simulink model "sysgen_oversample2x_2samples_per_clock"  (R2016b)
settings: Solver=VariableStepAuto  StartTime=0.0  StopTime=samples_per_channel*number_channels  RelTol=1e-3
PreLoadFcn:
  | setup
undefined symbols (not defined in the file or in its folder): j
libraries: xbsIndex_r4 x355, dspsigops x2, hdlsllib x2
(part 3 of 3)

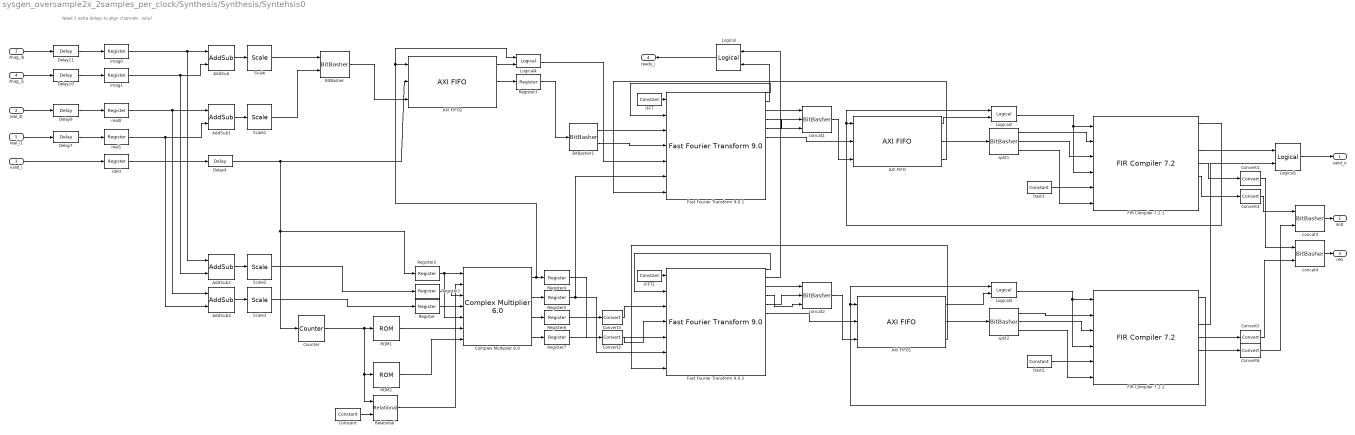
== system sysgen_oversample2x_2samples_per_clock/Synthesis/Synthesis/Syntehsis0 ==
  note: Need 2 extra delays to align channels - why?
  imag_i0 : Inport
  real_i0 : Inport  Port=2
  valid_i : Inport  Port=3
  imag_i1 : Inport  Port=4
  real_i1 : Inport  Port=5
  AXI FIFO : xbsIndex_r4/AXI FIFO  input_depth_axis=16  actual_fifo_depth_label=18  enable_tdata=on  enable_tdest=off  enable_tstrb=off  enable_tready=on  enable_tid=off  enable_tuser=off  enable_tkeep=off  enable_tlast=off  has_aresetn=off  enable_data_counts_axis=off  fifo_implementation_type_axis=Common Clock Block RAM  trim_axipin_name=on  programmable_full_type_axis=Full  full_threshold_assert_value_axis=0  programmable_empty_type_axis=Empty  empty_threshold_assert_value_axis=1022  underflow_flag_axi=0  underflow_sense_axi=Active High  overflow_flag_axi=0  overflow_sense_axi=Active High  block_type=axi_fifo
  AXI FIFO1 : xbsIndex_r4/AXI FIFO  input_depth_axis=16  actual_fifo_depth_label=18  enable_tdata=on  enable_tdest=off  enable_tstrb=off  enable_tready=on  enable_tid=off  enable_tuser=off  enable_tkeep=off  enable_tlast=off  has_aresetn=off  enable_data_counts_axis=off  fifo_implementation_type_axis=Common Clock Block RAM  trim_axipin_name=on  programmable_full_type_axis=Full  full_threshold_assert_value_axis=0  programmable_empty_type_axis=Empty  empty_threshold_assert_value_axis=1022  underflow_flag_axi=0  underflow_sense_axi=Active High  overflow_flag_axi=0  overflow_sense_axi=Active High  block_type=axi_fifo
  AXI FIFO2 : xbsIndex_r4/AXI FIFO  input_depth_axis=16  actual_fifo_depth_label=18  enable_tdata=on  enable_tdest=off  enable_tstrb=off  enable_tready=on  enable_tid=off  enable_tuser=off  enable_tkeep=off  enable_tlast=off  has_aresetn=off  enable_data_counts_axis=off  fifo_implementation_type_axis=Common Clock Block RAM  trim_axipin_name=on  programmable_full_type_axis=Full  full_threshold_assert_value_axis=0  programmable_empty_type_axis=Empty  empty_threshold_assert_value_axis=1022  underflow_flag_axi=0  underflow_sense_axi=Active High  overflow_flag_axi=0  overflow_sense_axi=Active High  block_type=axi_fifo
  AddSub : xbsIndex_r4/AddSub  mode=Addition  use_carryin=off  use_carryout=off  en=off  latency=2  precision=Full  arith_type="Signed  (2's comp)"  n_bits=17  bin_pt=15  quantization=Truncate  overflow=Saturate  use_behavioral_HDL=on  hw_selection=Fabric  pipelined=off  dbl_ovrd=off  block_type=addsub
  AddSub1 : xbsIndex_r4/AddSub  mode=Addition  use_carryin=off  use_carryout=off  en=off  latency=2  precision=Full  arith_type="Signed  (2's comp)"  n_bits=17  bin_pt=15  quantization=Truncate  overflow=Saturate  use_behavioral_HDL=on  hw_selection=Fabric  pipelined=off  dbl_ovrd=off  block_type=addsub
  AddSub2 : xbsIndex_r4/AddSub  mode=Subtraction  use_carryin=off  use_carryout=off  en=off  latency=2  precision=Full  arith_type="Signed  (2's comp)"  n_bits=17  bin_pt=15  quantization=Truncate  overflow=Saturate  use_behavioral_HDL=on  hw_selection=Fabric  pipelined=off  dbl_ovrd=off  block_type=addsub
  AddSub4 : xbsIndex_r4/AddSub  mode=Subtraction  use_carryin=off  use_carryout=off  en=off  latency=2  precision=Full  arith_type="Signed  (2's comp)"  n_bits=17  bin_pt=15  quantization=Truncate  overflow=Saturate  use_behavioral_HDL=on  hw_selection=Fabric  pipelined=off  dbl_ovrd=off  block_type=addsub
  BitBasher : xbsIndex_r4/BitBasher  bitexpr=out = {30'b0, im, re}  display_expr=off  sr_1=out  arith_type1=Unsigned  bin_pt1=0  sr_2=2  arith_type2=Unsigned  bin_pt2=0  sr_3=3  arith_type3=Unsigned  bin_pt3=0  sr_4=4  arith_type4=Unsigned  bin_pt4=0  dbl_ovrd=off  block_type=bitbasher
  BitBasher1 : xbsIndex_r4/BitBasher  bitexpr=|  display_expr=off  sr_1=im  arith_type1="Signed  (2's comp)"  bin_pt1=16  sr_2=re  arith_type2="Signed  (2's comp)"  bin_pt2=16  sr_3=3  arith_type3=Unsigned  bin_pt3=0  sr_4=4  arith_type4=Unsigned  bin_pt4=0  dbl_ovrd=off  block_type=bitbasher
      | im = {in[33:17]}
      | re = {in[16:0]}
  "Complex Multiplier 6.0 " : xbsIndex_r4/Complex Multiplier 6.0   hasatlast=on  hasatuser=off  atuserwidth=1  hasbtlast=off  hasbtuser=off  btuserwidth=1  multtype=Use_Mults  optimizegoal=Resources  flowcontrol=NonBlocking  outputwidth=19  roundmode=Truncate  hasctrltlast=off  hasctrltuser=off  ctrltuserwidth=1  outtlastbehv=Null  latencyconfig=Automatic  minimumlatency=37  aclken=off  aresetn=off  trim_axipin_name=on  simulation_type=hybrid_sim  simulation_model=sysgen:cmpy_v6_0  data_path_portlist={ 's_axis_a_tdata_real', 's_axis_a_tdata_imag', 's_axis_b_tdata_real', 's_axis_b_tdata_imag', 's_axis_ctrl_tdata_rounding_bit', 'm_axis_dout_tdata_real', 'm_axis_dout_tdata_imag' }  aportwidth=63  bportwidth=63  ip_name=Complex Multiplier  ip_version=6.0  dsptool_ready=true  ipcore_usecache=true  ipcore_useipmodelcache=true  ipcore_verbose=false  ipcore_latency_parameter='minimumlatency'  wrapper_available=true  port_translation_map={ 'aclken' => 'en', 'aresetn' => 'rst'}  block_type=cmpy_v6_0
  Constant : xbsIndex_r4/Constant  const=7  gui_display_data_type=Fixed-point  arith_type=Unsigned  n_bits=3  bin_pt=0  preci_type=Single  exp_width=8  frac_width=24  explicit_period=off  period=1  equ=P=C  opselect=C  inp2=PCIN>>17  opr=+  inp1=P  carry=CIN  dbl_ovrd=off  block_type=constant
  Convert{1,4..6} (4 alike) : xbsIndex_r4/Convert  gui_display_data_type=Fixed-point  arith_type="Signed  (2's comp)"  n_bits=16  bin_pt=15  float_type=Single  exp_bits=8  fraction_bits=24  quantization=Truncate  overflow=Wrap  en=off  latency=1  pipeline=off  dbl_ovrd=off  block_type=convert
  Convert2 : xbsIndex_r4/Convert  gui_display_data_type=Fixed-point  arith_type="Signed  (2's comp)"  n_bits=17  bin_pt=16  float_type=Single  exp_bits=8  fraction_bits=24  quantization=Truncate  overflow=Wrap  en=off  latency=0  pipeline=off  dbl_ovrd=off  block_type=convert
  Convert3 : xbsIndex_r4/Convert  gui_display_data_type=Fixed-point  arith_type="Signed  (2's comp)"  n_bits=17  bin_pt=16  float_type=Single  exp_bits=8  fraction_bits=24  quantization=Truncate  overflow=Wrap  en=off  latency=0  pipeline=off  dbl_ovrd=off  block_type=convert
  Counter : xbsIndex_r4/Counter  cnt_type=Free Running  cnt_to=Inf  operation=Up  start_count=0  cnt_by_val=1  arith_type=Unsigned  n_bits=3  bin_pt=0  load_pin=off  rst=off  en=on  explicit_period=on  period=2  use_behavioral_HDL=off  implementation=Fabric  dbl_ovrd=off  block_type=counter
  Delay{4,7,9..11} (5 alike) : xbsIndex_r4/Delay  rst=off  infoeditControl=Selection of Reset will increase slice count due to use of real FFs and instead of SRLs  en=off  latency=2  reg_retiming=off  dbl_ovrd=off  block_type=delay
  FIR Compiler 7.2 1 : xbsIndex_r4/FIR Compiler 7.2   coefficientvector=synthesis_coefficients1  coefficient_sets=8  coefficient_reload=off  filter_type=Single_Rate  rate_change_type=Integer  interpolation_rate=1  decimation_rate=1  zero_pack_factor=1  channel_sequence=Basic  number_channels=8  pattern_list='P4-0,P4-1,P4-2,P4-3,P4-4'  number_paths=2  ratespecification=Output_Sample_Period  sampleperiod=1  hardwareoversamplingrate=1  coefficient_sign=Signed  quantization=Quantize_Only  coefficient_width=25  bestprecision=on  coefficient_fractional_bits=28  coefficient_structure=Inferred  output_rounding_mode=Convergent_Rounding_to_Even  output_width=19  filter_architecture=Systolic_Multiply_Accumulate  optimization_goal=Area  optimization_list='None'  data_buffer_type=Automatic  coefficient_buffer_type=Automatic  input_buffer_type=Automatic  output_buffer_type=Automatic  preference_for_other_storage=Automatic  multi_column_support=Automatic  columnconfig='16'  inter_column_pipe_length=4  data_has_tlast=Not_Required  m_data_has_tready=off  s_data_has_fifo=off  s_data_has_tuser=Not_Required  m_data_has_tuser=Not_Required  s_config_sync_mode=On_Vector  s_config_method=By_Channel  num_reload_slots=1  has_aclken=off  has_aresetn=off  infoeditControl=ARESETn must be asserted for a minimum of 2 cycles  reset_data_vector=on  trim_axipin_name=on  simulation_type=hybrid_sim  simulation_model=sysgen:xfirv7_2_cmodel  data_path_portlist={ 's_axis_data_tdata', 'm_axis_data_tdata' }  passband_min=0.0  passband_max=0.5  stopband_min=0.5  stopband_max=1.0  filter_selection=1  gui_behaviour='Sysgen_GUI'  data_sign=Signed  data_width=16  data_fractional_bits=0  data_tuser_width=1  wrapper_available=true  ip_wrap_arbitrary_binary_point=true  ip_name=FIR Compiler  ip_version=7.2  dsptool_ready=true  ipcore_usecache=true  ipcore_useipmodelcache=true  port_translation_map={ 'aclken' => 'en', 'aresetn' => 'rst' }  run_core_at_system_period=true  ipcore_xco_need_fpga_part=true  block_type=fir_compiler_v7_2
      settings: infoedit=Maximum Possible : Maximizes oversampling rate. Abstracted input handshake (no s_data_tvalid) and automatic rate propagation.<br>Hardware Oversampling Rate : Specifies oversampling rate relative to the input sample period. Abstracted input handshake (no s_data_tvalid) and automatic rate propagation.<br>Input/Output Sample Period : Specifies absolute oversampling rate. No input handshake abstraction (exposes s_data_tvalid) and no rate propagation.
  FIR Compiler 7.2 2 : xbsIndex_r4/FIR Compiler 7.2   coefficientvector=synthesis_coefficients2  coefficient_sets=8  coefficient_reload=off  filter_type=Single_Rate  rate_change_type=Integer  interpolation_rate=1  decimation_rate=1  zero_pack_factor=1  channel_sequence=Basic  number_channels=8  pattern_list='P4-0,P4-1,P4-2,P4-3,P4-4'  number_paths=2  ratespecification=Output_Sample_Period  sampleperiod=1  hardwareoversamplingrate=1  coefficient_sign=Signed  quantization=Quantize_Only  coefficient_width=25  bestprecision=on  coefficient_fractional_bits=28  coefficient_structure=Inferred  output_rounding_mode=Convergent_Rounding_to_Even  output_width=19  filter_architecture=Systolic_Multiply_Accumulate  optimization_goal=Area  optimization_list='None'  data_buffer_type=Automatic  coefficient_buffer_type=Automatic  input_buffer_type=Automatic  output_buffer_type=Automatic  preference_for_other_storage=Automatic  multi_column_support=Automatic  columnconfig='16'  inter_column_pipe_length=4  data_has_tlast=Not_Required  m_data_has_tready=off  s_data_has_fifo=off  s_data_has_tuser=Not_Required  m_data_has_tuser=Not_Required  s_config_sync_mode=On_Vector  s_config_method=By_Channel  num_reload_slots=1  has_aclken=off  has_aresetn=off  infoeditControl=ARESETn must be asserted for a minimum of 2 cycles  reset_data_vector=on  trim_axipin_name=on  simulation_type=hybrid_sim  simulation_model=sysgen:xfirv7_2_cmodel  data_path_portlist={ 's_axis_data_tdata', 'm_axis_data_tdata' }  passband_min=0.0  passband_max=0.5  stopband_min=0.5  stopband_max=1.0  filter_selection=1  gui_behaviour='Sysgen_GUI'  data_sign=Signed  data_width=16  data_fractional_bits=0  data_tuser_width=1  wrapper_available=true  ip_wrap_arbitrary_binary_point=true  ip_name=FIR Compiler  ip_version=7.2  dsptool_ready=true  ipcore_usecache=true  ipcore_useipmodelcache=true  port_translation_map={ 'aclken' => 'en', 'aresetn' => 'rst' }  run_core_at_system_period=true  ipcore_xco_need_fpga_part=true  block_type=fir_compiler_v7_2
      settings: infoedit=Maximum Possible : Maximizes oversampling rate. Abstracted input handshake (no s_data_tvalid) and automatic rate propagation.<br>Hardware Oversampling Rate : Specifies oversampling rate relative to the input sample period. Abstracted input handshake (no s_data_tvalid) and automatic rate propagation.<br>Input/Output Sample Period : Specifies absolute oversampling rate. No input handshake abstraction (exposes s_data_tvalid) and no rate propagation.
  Fast Fourier Transform 9.0 1 : xbsIndex_r4/Fast Fourier Transform 9.0   transform_length=8  target_clock_frequency=250  target_data_throughput=50  implementation_options=pipelined_streaming_io  run_time_configurable_transform_length=off  phase_factor_width=17  scaling_options=unscaled  rounding_modes=convergent_rounding  aclken=off  aresetn=off  output_ordering=natural_order  cyclic_prefix_insertion=off  throttle_scheme=nonrealtime  xk_index=on  ovflo=off  trim_axipin_name=on  memory_options_data=block_ram  memory_options_phase_factors=block_ram  number_of_stages_using_block_ram_for_data_and_phase_factors=0  memory_options_reorder=block_ram  memory_options_hybrid=off  complex_mult_type=use_mults_resources  butterfly_type=use_xtremedsp_slices  simulation_type=hybrid_sim  simulation_model=sysgen:xfftv9_cmodel  data_path_portlist={ 's_axis_data_tdata', 'm_axis_data_tdata', 'm_axis_status_tdata', 'event_fft_overflow' }  channels=1  input_ordering=natural_order  input_width=16  ip_name=Fast Fourier Transform  ip_version=9.0  dsptool_ready=true  ipcore_usecache=true  ipcore_useipmodelcache=true  wrapper_available=true  port_translation_map={ 'aclken' => 'en', 'aresetn' => 'rst'}  data_format=fixed_point  block_type=xfft_v9_0
  Fast Fourier Transform 9.0 2 : xbsIndex_r4/Fast Fourier Transform 9.0   transform_length=8  target_clock_frequency=250  target_data_throughput=50  implementation_options=pipelined_streaming_io  run_time_configurable_transform_length=off  phase_factor_width=17  scaling_options=unscaled  rounding_modes=convergent_rounding  aclken=off  aresetn=off  output_ordering=natural_order  cyclic_prefix_insertion=off  throttle_scheme=nonrealtime  xk_index=on  ovflo=off  trim_axipin_name=on  memory_options_data=block_ram  memory_options_phase_factors=block_ram  number_of_stages_using_block_ram_for_data_and_phase_factors=0  memory_options_reorder=block_ram  memory_options_hybrid=off  complex_mult_type=use_mults_resources  butterfly_type=use_xtremedsp_slices  simulation_type=hybrid_sim  simulation_model=sysgen:xfftv9_cmodel  data_path_portlist={ 's_axis_data_tdata', 'm_axis_data_tdata', 'm_axis_status_tdata', 'event_fft_overflow' }  channels=1  input_ordering=natural_order  input_width=16  ip_name=Fast Fourier Transform  ip_version=9.0  dsptool_ready=true  ipcore_usecache=true  ipcore_useipmodelcache=true  wrapper_available=true  port_translation_map={ 'aclken' => 'en', 'aresetn' => 'rst'}  data_format=fixed_point  block_type=xfft_v9_0
  IFFT : xbsIndex_r4/Constant  const=0  gui_display_data_type=Fixed-point  arith_type=Unsigned  n_bits=1  bin_pt=0  preci_type=Single  exp_width=8  frac_width=24  explicit_period=off  period=1  equ=P=C  opselect=C  inp2=PCIN>>17  opr=+  inp1=P  carry=CIN  dbl_ovrd=off  block_type=constant
  IFFT1 : xbsIndex_r4/Constant  const=0  gui_display_data_type=Fixed-point  arith_type=Unsigned  n_bits=1  bin_pt=0  preci_type=Single  exp_width=8  frac_width=24  explicit_period=off  period=1  equ=P=C  opselect=C  inp2=PCIN>>17  opr=+  inp1=P  carry=CIN  dbl_ovrd=off  block_type=constant
  Logical : xbsIndex_r4/Logical  logical_function=AND  inputs=2  en=off  latency=1  precision=Full  arith_type=Unsigned  n_bits=16  bin_pt=0  align_bp=on  dbl_ovrd=off  block_type=logical
  Logical1 : xbsIndex_r4/Logical  logical_function=AND  inputs=2  en=off  latency=1  precision=Full  arith_type=Unsigned  n_bits=16  bin_pt=0  align_bp=on  dbl_ovrd=off  block_type=logical
  Logical2 : xbsIndex_r4/Logical  logical_function=AND  inputs=2  en=off  latency=0  precision=Full  arith_type=Unsigned  n_bits=16  bin_pt=0  align_bp=on  dbl_ovrd=off  block_type=logical
  Logical3 : xbsIndex_r4/Logical  logical_function=AND  inputs=2  en=off  latency=0  precision=Full  arith_type=Unsigned  n_bits=16  bin_pt=0  align_bp=on  dbl_ovrd=off  block_type=logical
  Logical4 : xbsIndex_r4/Logical  logical_function=AND  inputs=2  en=off  latency=1  precision=Full  arith_type=Unsigned  n_bits=16  bin_pt=0  align_bp=on  dbl_ovrd=off  block_type=logical
  ROM1 : xbsIndex_r4/ROM  depth=8  initVector=imag(exp(j*2*pi*(0:7)/16))  distributed_mem=Block RAM  rst=off  init_reg=0  en=off  latency=1  gui_display_data_type=Fixed-point  arith_type="Signed  (2's comp)"  n_bits=18  bin_pt=17  preci_type=Single  exp_width=8  frac_width=24  optimize=Area  use_rpm=on  dbl_ovrd=off  block_type=sprom
  ROM2 : xbsIndex_r4/ROM  depth=8  initVector=real(exp(j*2*pi*(0:7)/16))  distributed_mem=Block RAM  rst=off  init_reg=0  en=off  latency=1  gui_display_data_type=Fixed-point  arith_type="Signed  (2's comp)"  n_bits=18  bin_pt=17  preci_type=Single  exp_width=8  frac_width=24  optimize=Area  use_rpm=on  dbl_ovrd=off  block_type=sprom
  Register{,1..7} (8 alike) : xbsIndex_r4/Register  init=0  rst=off  en=off  dbl_ovrd=off  block_type=register
  Relational : xbsIndex_r4/Relational  mode=a=b  op_type=Bool  en=off  latency=1  dbl_ovrd=off  block_type=relational
  Scale{,1..3} (4 alike) : xbsIndex_r4/Scale  scale_factor=-1  dbl_ovrd=off  block_type=scale
  concat1 : xbsIndex_r4/BitBasher  bitexpr=o={21'b0,index, im[19:0], re[19:0] }  display_expr=off  sr_1=o  arith_type1=Unsigned  bin_pt1=0  sr_2=2  arith_type2=Unsigned  bin_pt2=0  sr_3=3  arith_type3=Unsigned  bin_pt3=0  sr_4=4  arith_type4=Unsigned  bin_pt4=0  dbl_ovrd=off  block_type=bitbasher
  concat2 : xbsIndex_r4/BitBasher  bitexpr=o={21'b0,index, im[19:0], re[19:0] }  display_expr=off  sr_1=o  arith_type1=Unsigned  bin_pt1=0  sr_2=2  arith_type2=Unsigned  bin_pt2=0  sr_3=3  arith_type3=Unsigned  bin_pt3=0  sr_4=4  arith_type4=Unsigned  bin_pt4=0  dbl_ovrd=off  block_type=bitbasher
  concat3 : xbsIndex_r4/BitBasher  bitexpr=o={hi,low }  display_expr=off  sr_1=o  arith_type1=Unsigned  bin_pt1=0  sr_2=2  arith_type2=Unsigned  bin_pt2=0  sr_3=3  arith_type3=Unsigned  bin_pt3=0  sr_4=4  arith_type4=Unsigned  bin_pt4=0  dbl_ovrd=off  block_type=bitbasher
  concat4 : xbsIndex_r4/BitBasher  bitexpr=o={hi,low }  display_expr=off  sr_1=o  arith_type1=Unsigned  bin_pt1=0  sr_2=2  arith_type2=Unsigned  bin_pt2=0  sr_3=3  arith_type3=Unsigned  bin_pt3=0  sr_4=4  arith_type4=Unsigned  bin_pt4=0  dbl_ovrd=off  block_type=bitbasher
  imag0 : xbsIndex_r4/Register  init=0  rst=off  en=off  dbl_ovrd=off  block_type=register
  imag1 : xbsIndex_r4/Register  init=0  rst=off  en=off  dbl_ovrd=off  block_type=register
  real0 : xbsIndex_r4/Register  init=0  rst=off  en=off  dbl_ovrd=off  block_type=register
  real1 : xbsIndex_r4/Register  init=0  rst=off  en=off  dbl_ovrd=off  block_type=register
  split1 : xbsIndex_r4/BitBasher  bitexpr=|  display_expr=off  sr_1=re  arith_type1="Signed  (2's comp)"  bin_pt1=13  sr_2=im  arith_type2="Signed  (2's comp)"  bin_pt2=13  sr_3=index  arith_type3=Unsigned  bin_pt3=0  sr_4=4  arith_type4=Unsigned  bin_pt4=0  dbl_ovrd=off  block_type=bitbasher
      | re={in[19:2]}
      | im={in[39:22]}
      | index = {in[42:40]}
  split2 : xbsIndex_r4/BitBasher  bitexpr=|  display_expr=off  sr_1=re  arith_type1="Signed  (2's comp)"  bin_pt1=13  sr_2=im  arith_type2="Signed  (2's comp)"  bin_pt2=13  sr_3=index  arith_type3=Unsigned  bin_pt3=0  sr_4=4  arith_type4=Unsigned  bin_pt4=0  dbl_ovrd=off  block_type=bitbasher
      | re={in[19:2]}
      | im={in[39:22]}
      | index = {in[42:40]}
  tlast2 : xbsIndex_r4/Constant  const=0  gui_display_data_type=Boolean  arith_type=Boolean  n_bits=8  bin_pt=0  preci_type=Single  exp_width=8  frac_width=24  explicit_period=off  period=1  equ=P=C  opselect=C  inp2=PCIN>>17  opr=+  inp1=P  carry=CIN  dbl_ovrd=off  block_type=constant
  tlast3 : xbsIndex_r4/Constant  const=0  gui_display_data_type=Boolean  arith_type=Boolean  n_bits=8  bin_pt=0  preci_type=Single  exp_width=8  frac_width=24  explicit_period=off  period=1  equ=P=C  opselect=C  inp2=PCIN>>17  opr=+  inp1=P  carry=CIN  dbl_ovrd=off  block_type=constant
  valid : xbsIndex_r4/Register  init=0  rst=off  en=off  dbl_ovrd=off  block_type=register
  valid_o : Outport
  im0 : Outport  Port=2
  re0 : Outport  Port=3
  ready_i : Outport  Port=4
  wires:
  concat3/1 -> im0/1
  Convert6/1 -> concat3/2
  Convert4/1 -> concat3/1
  concat4/1 -> re0/1
  IFFT/1 -> Fast Fourier Transform 9.0 1/1
  Fast Fourier Transform 9.0 1/3 -> concat1/1
  concat1/1 -> AXI FIFO/3
  AXI FIFO/3 -> Fast Fourier Transform 9.0 1/7
  IFFT1/1 -> Fast Fourier Transform 9.0 2/1
  Convert3/1 -> Fast Fourier Transform 9.0 2/3
  Register2/1 -> "Complex Multiplier 6.0 "/1, "Complex Multiplier 6.0 "/5
  AXI FIFO1/2 -> split2/1
  FIR Compiler 7.2 1/1 -> Logical2/1, AXI FIFO/1
  split2/1 -> FIR Compiler 7.2 2/2
  FIR Compiler 7.2 2/1 -> Logical3/1, AXI FIFO1/1
  AddSub1/1 -> Scale1/1
  Fast Fourier Transform 9.0 1/2 -> Logical/2
  Fast Fourier Transform 9.0 2/2 -> Logical/1
  Logical/1 -> ready_i/1
  real0/1 -> AddSub4/1, AddSub1/1
  imag1/1 -> AddSub2/2, AddSub/2
  real1/1 -> AddSub4/2, AddSub1/2
  valid/1 -> Delay4/1
  imag0/1 -> AddSub2/1, AddSub/1
  AddSub4/1 -> Scale3/1
  AddSub2/1 -> Scale2/1
  FIR Compiler 7.2 1/3 -> Logical1/1
  FIR Compiler 7.2 2/3 -> Logical1/2
  Logical1/1 -> valid_o/1
  Counter/1 -> ROM2/1, Relational/1, ROM1/1
  Convert2/1 -> Fast Fourier Transform 9.0 2/4
  "Complex Multiplier 6.0 "/1 -> Register4/1, AXI FIFO2/1, Logical4/1
  Delay4/1 -> AXI FIFO2/2, Counter/1, Register2/1
  Fast Fourier Transform 9.0 1/6 -> AXI FIFO/2
  Fast Fourier Transform 9.0 1/4 -> concat1/3
  Fast Fourier Transform 9.0 2/3 -> concat2/1
  Fast Fourier Transform 9.0 2/5 -> concat2/2
  Fast Fourier Transform 9.0 2/6 -> AXI FIFO1/2
  concat2/1 -> AXI FIFO1/3
  AXI FIFO/2 -> split1/1
  Fast Fourier Transform 9.0 1/5 -> concat1/2
  AddSub/1 -> Scale/1
  AXI FIFO/1 -> Logical2/2
  AXI FIFO1/1 -> Logical3/2
  FIR Compiler 7.2 1/4 -> Convert1/1
  FIR Compiler 7.2 1/5 -> Convert4/1
  FIR Compiler 7.2 2/4 -> Convert5/1
  FIR Compiler 7.2 2/5 -> Convert6/1
  split1/1 -> FIR Compiler 7.2 1/2
  Fast Fourier Transform 9.0 2/4 -> concat2/3
  split2/2 -> FIR Compiler 7.2 2/3
  Logical3/1 -> FIR Compiler 7.2 2/4, FIR Compiler 7.2 2/1
  split1/2 -> FIR Compiler 7.2 1/3
  Logical2/1 -> FIR Compiler 7.2 1/4, FIR Compiler 7.2 1/1
  tlast2/1 -> FIR Compiler 7.2 2/5
  tlast3/1 -> FIR Compiler 7.2 1/5
  split2/3 -> FIR Compiler 7.2 2/6
  split1/3 -> FIR Compiler 7.2 1/6
  imag_i0/1 -> Delay11/1
  imag_i1/1 -> Delay10/1
  real_i0/1 -> Delay9/1
  real_i1/1 -> Delay7/1
  valid_i/1 -> valid/1
  Scale2/1 -> Register1/1
  Scale3/1 -> Register/1
  "Complex Multiplier 6.0 "/3 -> Register6/1
  "Complex Multiplier 6.0 "/4 -> Register7/1
  Register/1 -> "Complex Multiplier 6.0 "/4
  Register1/1 -> "Complex Multiplier 6.0 "/3
  ROM2/1 -> "Complex Multiplier 6.0 "/7
  ROM1/1 -> "Complex Multiplier 6.0 "/6
  Relational/1 -> "Complex Multiplier 6.0 "/2
  Constant/1 -> Relational/2
  "Complex Multiplier 6.0 "/2 -> Register5/1
  Fast Fourier Transform 9.0 2/1 -> Fast Fourier Transform 9.0 2/2
  Fast Fourier Transform 9.0 1/1 -> Fast Fourier Transform 9.0 1/2
  AXI FIFO1/3 -> Fast Fourier Transform 9.0 2/7
  Delay7/1 -> real1/1
  Delay9/1 -> real0/1
  Delay10/1 -> imag1/1
  Delay11/1 -> imag0/1
  Scale/1 -> BitBasher/1
  Scale1/1 -> BitBasher/2
  BitBasher/1 -> AXI FIFO2/3
  AXI FIFO2/1 -> Logical4/2
  BitBasher1/1 -> Fast Fourier Transform 9.0 1/3
  BitBasher1/2 -> Fast Fourier Transform 9.0 1/4
  AXI FIFO2/2 -> Register3/1
  Register3/1 -> BitBasher1/1
  Logical4/1 -> Fast Fourier Transform 9.0 1/5
  Register4/1 -> Fast Fourier Transform 9.0 2/5
  Register5/1 -> Fast Fourier Transform 9.0 1/6, Fast Fourier Transform 9.0 2/6
  Register6/1 -> Convert3/1
  Register7/1 -> Convert2/1
  Convert1/1 -> concat4/1
  Convert5/1 -> concat4/2

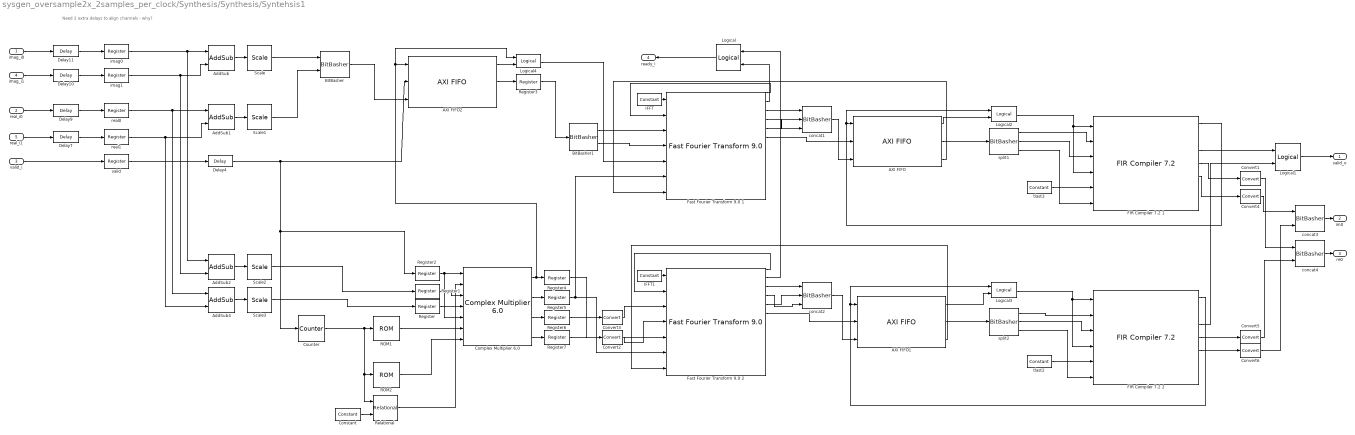
== system sysgen_oversample2x_2samples_per_clock/Synthesis/Synthesis/Syntehsis1 ==
  note: Need 2 extra delays to align channels - why?
  imag_i0 : Inport
  real_i0 : Inport  Port=2
  valid_i : Inport  Port=3
  imag_i1 : Inport  Port=4
  real_i1 : Inport  Port=5
  AXI FIFO : xbsIndex_r4/AXI FIFO  input_depth_axis=16  actual_fifo_depth_label=18  enable_tdata=on  enable_tdest=off  enable_tstrb=off  enable_tready=on  enable_tid=off  enable_tuser=off  enable_tkeep=off  enable_tlast=off  has_aresetn=off  enable_data_counts_axis=off  fifo_implementation_type_axis=Common Clock Block RAM  trim_axipin_name=on  programmable_full_type_axis=Full  full_threshold_assert_value_axis=0  programmable_empty_type_axis=Empty  empty_threshold_assert_value_axis=1022  underflow_flag_axi=0  underflow_sense_axi=Active High  overflow_flag_axi=0  overflow_sense_axi=Active High  block_type=axi_fifo
  AXI FIFO1 : xbsIndex_r4/AXI FIFO  input_depth_axis=16  actual_fifo_depth_label=18  enable_tdata=on  enable_tdest=off  enable_tstrb=off  enable_tready=on  enable_tid=off  enable_tuser=off  enable_tkeep=off  enable_tlast=off  has_aresetn=off  enable_data_counts_axis=off  fifo_implementation_type_axis=Common Clock Block RAM  trim_axipin_name=on  programmable_full_type_axis=Full  full_threshold_assert_value_axis=0  programmable_empty_type_axis=Empty  empty_threshold_assert_value_axis=1022  underflow_flag_axi=0  underflow_sense_axi=Active High  overflow_flag_axi=0  overflow_sense_axi=Active High  block_type=axi_fifo
  AXI FIFO2 : xbsIndex_r4/AXI FIFO  input_depth_axis=16  actual_fifo_depth_label=18  enable_tdata=on  enable_tdest=off  enable_tstrb=off  enable_tready=on  enable_tid=off  enable_tuser=off  enable_tkeep=off  enable_tlast=off  has_aresetn=off  enable_data_counts_axis=off  fifo_implementation_type_axis=Common Clock Block RAM  trim_axipin_name=on  programmable_full_type_axis=Full  full_threshold_assert_value_axis=0  programmable_empty_type_axis=Empty  empty_threshold_assert_value_axis=1022  underflow_flag_axi=0  underflow_sense_axi=Active High  overflow_flag_axi=0  overflow_sense_axi=Active High  block_type=axi_fifo
  AddSub : xbsIndex_r4/AddSub  mode=Addition  use_carryin=off  use_carryout=off  en=off  latency=2  precision=Full  arith_type="Signed  (2's comp)"  n_bits=17  bin_pt=15  quantization=Truncate  overflow=Saturate  use_behavioral_HDL=on  hw_selection=Fabric  pipelined=off  dbl_ovrd=off  block_type=addsub
  AddSub1 : xbsIndex_r4/AddSub  mode=Addition  use_carryin=off  use_carryout=off  en=off  latency=2  precision=Full  arith_type="Signed  (2's comp)"  n_bits=17  bin_pt=15  quantization=Truncate  overflow=Saturate  use_behavioral_HDL=on  hw_selection=Fabric  pipelined=off  dbl_ovrd=off  block_type=addsub
  AddSub2 : xbsIndex_r4/AddSub  mode=Subtraction  use_carryin=off  use_carryout=off  en=off  latency=2  precision=Full  arith_type="Signed  (2's comp)"  n_bits=17  bin_pt=15  quantization=Truncate  overflow=Saturate  use_behavioral_HDL=on  hw_selection=Fabric  pipelined=off  dbl_ovrd=off  block_type=addsub
  AddSub4 : xbsIndex_r4/AddSub  mode=Subtraction  use_carryin=off  use_carryout=off  en=off  latency=2  precision=Full  arith_type="Signed  (2's comp)"  n_bits=17  bin_pt=15  quantization=Truncate  overflow=Saturate  use_behavioral_HDL=on  hw_selection=Fabric  pipelined=off  dbl_ovrd=off  block_type=addsub
  BitBasher : xbsIndex_r4/BitBasher  bitexpr=out = {30'b0, im, re}  display_expr=off  sr_1=out  arith_type1=Unsigned  bin_pt1=0  sr_2=2  arith_type2=Unsigned  bin_pt2=0  sr_3=3  arith_type3=Unsigned  bin_pt3=0  sr_4=4  arith_type4=Unsigned  bin_pt4=0  dbl_ovrd=off  block_type=bitbasher
  BitBasher1 : xbsIndex_r4/BitBasher  bitexpr=|  display_expr=off  sr_1=im  arith_type1="Signed  (2's comp)"  bin_pt1=16  sr_2=re  arith_type2="Signed  (2's comp)"  bin_pt2=16  sr_3=3  arith_type3=Unsigned  bin_pt3=0  sr_4=4  arith_type4=Unsigned  bin_pt4=0  dbl_ovrd=off  block_type=bitbasher
      | im = {in[33:17]}
      | re = {in[16:0]}
  "Complex Multiplier 6.0 " : xbsIndex_r4/Complex Multiplier 6.0   hasatlast=on  hasatuser=off  atuserwidth=1  hasbtlast=off  hasbtuser=off  btuserwidth=1  multtype=Use_Mults  optimizegoal=Resources  flowcontrol=NonBlocking  outputwidth=19  roundmode=Truncate  hasctrltlast=off  hasctrltuser=off  ctrltuserwidth=1  outtlastbehv=Null  latencyconfig=Automatic  minimumlatency=37  aclken=off  aresetn=off  trim_axipin_name=on  simulation_type=hybrid_sim  simulation_model=sysgen:cmpy_v6_0  data_path_portlist={ 's_axis_a_tdata_real', 's_axis_a_tdata_imag', 's_axis_b_tdata_real', 's_axis_b_tdata_imag', 's_axis_ctrl_tdata_rounding_bit', 'm_axis_dout_tdata_real', 'm_axis_dout_tdata_imag' }  aportwidth=63  bportwidth=63  ip_name=Complex Multiplier  ip_version=6.0  dsptool_ready=true  ipcore_usecache=true  ipcore_useipmodelcache=true  ipcore_verbose=false  ipcore_latency_parameter='minimumlatency'  wrapper_available=true  port_translation_map={ 'aclken' => 'en', 'aresetn' => 'rst'}  block_type=cmpy_v6_0
  Constant : xbsIndex_r4/Constant  const=7  gui_display_data_type=Fixed-point  arith_type=Unsigned  n_bits=3  bin_pt=0  preci_type=Single  exp_width=8  frac_width=24  explicit_period=off  period=1  equ=P=C  opselect=C  inp2=PCIN>>17  opr=+  inp1=P  carry=CIN  dbl_ovrd=off  block_type=constant
  Convert{1,4..6} (4 alike) : xbsIndex_r4/Convert  gui_display_data_type=Fixed-point  arith_type="Signed  (2's comp)"  n_bits=16  bin_pt=15  float_type=Single  exp_bits=8  fraction_bits=24  quantization=Truncate  overflow=Wrap  en=off  latency=1  pipeline=off  dbl_ovrd=off  block_type=convert
  Convert2 : xbsIndex_r4/Convert  gui_display_data_type=Fixed-point  arith_type="Signed  (2's comp)"  n_bits=17  bin_pt=16  float_type=Single  exp_bits=8  fraction_bits=24  quantization=Truncate  overflow=Wrap  en=off  latency=0  pipeline=off  dbl_ovrd=off  block_type=convert
  Convert3 : xbsIndex_r4/Convert  gui_display_data_type=Fixed-point  arith_type="Signed  (2's comp)"  n_bits=17  bin_pt=16  float_type=Single  exp_bits=8  fraction_bits=24  quantization=Truncate  overflow=Wrap  en=off  latency=0  pipeline=off  dbl_ovrd=off  block_type=convert
  Counter : xbsIndex_r4/Counter  cnt_type=Free Running  cnt_to=Inf  operation=Up  start_count=0  cnt_by_val=1  arith_type=Unsigned  n_bits=3  bin_pt=0  load_pin=off  rst=off  en=on  explicit_period=on  period=2  use_behavioral_HDL=off  implementation=Fabric  dbl_ovrd=off  block_type=counter
  Delay{4,7,9..11} (5 alike) : xbsIndex_r4/Delay  rst=off  infoeditControl=Selection of Reset will increase slice count due to use of real FFs and instead of SRLs  en=off  latency=2  reg_retiming=off  dbl_ovrd=off  block_type=delay
  FIR Compiler 7.2 1 : xbsIndex_r4/FIR Compiler 7.2   coefficientvector=synthesis_coefficients1  coefficient_sets=8  coefficient_reload=off  filter_type=Single_Rate  rate_change_type=Integer  interpolation_rate=1  decimation_rate=1  zero_pack_factor=1  channel_sequence=Basic  number_channels=8  pattern_list='P4-0,P4-1,P4-2,P4-3,P4-4'  number_paths=2  ratespecification=Output_Sample_Period  sampleperiod=1  hardwareoversamplingrate=1  coefficient_sign=Signed  quantization=Quantize_Only  coefficient_width=25  bestprecision=on  coefficient_fractional_bits=28  coefficient_structure=Inferred  output_rounding_mode=Convergent_Rounding_to_Even  output_width=19  filter_architecture=Systolic_Multiply_Accumulate  optimization_goal=Area  optimization_list='None'  data_buffer_type=Automatic  coefficient_buffer_type=Automatic  input_buffer_type=Automatic  output_buffer_type=Automatic  preference_for_other_storage=Automatic  multi_column_support=Automatic  columnconfig='16'  inter_column_pipe_length=4  data_has_tlast=Not_Required  m_data_has_tready=off  s_data_has_fifo=off  s_data_has_tuser=Not_Required  m_data_has_tuser=Not_Required  s_config_sync_mode=On_Vector  s_config_method=By_Channel  num_reload_slots=1  has_aclken=off  has_aresetn=off  infoeditControl=ARESETn must be asserted for a minimum of 2 cycles  reset_data_vector=on  trim_axipin_name=on  simulation_type=hybrid_sim  simulation_model=sysgen:xfirv7_2_cmodel  data_path_portlist={ 's_axis_data_tdata', 'm_axis_data_tdata' }  passband_min=0.0  passband_max=0.5  stopband_min=0.5  stopband_max=1.0  filter_selection=1  gui_behaviour='Sysgen_GUI'  data_sign=Signed  data_width=16  data_fractional_bits=0  data_tuser_width=1  wrapper_available=true  ip_wrap_arbitrary_binary_point=true  ip_name=FIR Compiler  ip_version=7.2  dsptool_ready=true  ipcore_usecache=true  ipcore_useipmodelcache=true  port_translation_map={ 'aclken' => 'en', 'aresetn' => 'rst' }  run_core_at_system_period=true  ipcore_xco_need_fpga_part=true  block_type=fir_compiler_v7_2
      settings: infoedit=Maximum Possible : Maximizes oversampling rate. Abstracted input handshake (no s_data_tvalid) and automatic rate propagation.<br>Hardware Oversampling Rate : Specifies oversampling rate relative to the input sample period. Abstracted input handshake (no s_data_tvalid) and automatic rate propagation.<br>Input/Output Sample Period : Specifies absolute oversampling rate. No input handshake abstraction (exposes s_data_tvalid) and no rate propagation.
  FIR Compiler 7.2 2 : xbsIndex_r4/FIR Compiler 7.2   coefficientvector=synthesis_coefficients2  coefficient_sets=8  coefficient_reload=off  filter_type=Single_Rate  rate_change_type=Integer  interpolation_rate=1  decimation_rate=1  zero_pack_factor=1  channel_sequence=Basic  number_channels=8  pattern_list='P4-0,P4-1,P4-2,P4-3,P4-4'  number_paths=2  ratespecification=Output_Sample_Period  sampleperiod=1  hardwareoversamplingrate=1  coefficient_sign=Signed  quantization=Quantize_Only  coefficient_width=25  bestprecision=on  coefficient_fractional_bits=28  coefficient_structure=Inferred  output_rounding_mode=Convergent_Rounding_to_Even  output_width=19  filter_architecture=Systolic_Multiply_Accumulate  optimization_goal=Area  optimization_list='None'  data_buffer_type=Automatic  coefficient_buffer_type=Automatic  input_buffer_type=Automatic  output_buffer_type=Automatic  preference_for_other_storage=Automatic  multi_column_support=Automatic  columnconfig='16'  inter_column_pipe_length=4  data_has_tlast=Not_Required  m_data_has_tready=off  s_data_has_fifo=off  s_data_has_tuser=Not_Required  m_data_has_tuser=Not_Required  s_config_sync_mode=On_Vector  s_config_method=By_Channel  num_reload_slots=1  has_aclken=off  has_aresetn=off  infoeditControl=ARESETn must be asserted for a minimum of 2 cycles  reset_data_vector=on  trim_axipin_name=on  simulation_type=hybrid_sim  simulation_model=sysgen:xfirv7_2_cmodel  data_path_portlist={ 's_axis_data_tdata', 'm_axis_data_tdata' }  passband_min=0.0  passband_max=0.5  stopband_min=0.5  stopband_max=1.0  filter_selection=1  gui_behaviour='Sysgen_GUI'  data_sign=Signed  data_width=16  data_fractional_bits=0  data_tuser_width=1  wrapper_available=true  ip_wrap_arbitrary_binary_point=true  ip_name=FIR Compiler  ip_version=7.2  dsptool_ready=true  ipcore_usecache=true  ipcore_useipmodelcache=true  port_translation_map={ 'aclken' => 'en', 'aresetn' => 'rst' }  run_core_at_system_period=true  ipcore_xco_need_fpga_part=true  block_type=fir_compiler_v7_2
      settings: infoedit=Maximum Possible : Maximizes oversampling rate. Abstracted input handshake (no s_data_tvalid) and automatic rate propagation.<br>Hardware Oversampling Rate : Specifies oversampling rate relative to the input sample period. Abstracted input handshake (no s_data_tvalid) and automatic rate propagation.<br>Input/Output Sample Period : Specifies absolute oversampling rate. No input handshake abstraction (exposes s_data_tvalid) and no rate propagation.
  Fast Fourier Transform 9.0 1 : xbsIndex_r4/Fast Fourier Transform 9.0   transform_length=8  target_clock_frequency=250  target_data_throughput=50  implementation_options=pipelined_streaming_io  run_time_configurable_transform_length=off  phase_factor_width=17  scaling_options=unscaled  rounding_modes=convergent_rounding  aclken=off  aresetn=off  output_ordering=natural_order  cyclic_prefix_insertion=off  throttle_scheme=nonrealtime  xk_index=on  ovflo=off  trim_axipin_name=on  memory_options_data=block_ram  memory_options_phase_factors=block_ram  number_of_stages_using_block_ram_for_data_and_phase_factors=0  memory_options_reorder=block_ram  memory_options_hybrid=off  complex_mult_type=use_mults_resources  butterfly_type=use_xtremedsp_slices  simulation_type=hybrid_sim  simulation_model=sysgen:xfftv9_cmodel  data_path_portlist={ 's_axis_data_tdata', 'm_axis_data_tdata', 'm_axis_status_tdata', 'event_fft_overflow' }  channels=1  input_ordering=natural_order  input_width=16  ip_name=Fast Fourier Transform  ip_version=9.0  dsptool_ready=true  ipcore_usecache=true  ipcore_useipmodelcache=true  wrapper_available=true  port_translation_map={ 'aclken' => 'en', 'aresetn' => 'rst'}  data_format=fixed_point  block_type=xfft_v9_0
  Fast Fourier Transform 9.0 2 : xbsIndex_r4/Fast Fourier Transform 9.0   transform_length=8  target_clock_frequency=250  target_data_throughput=50  implementation_options=pipelined_streaming_io  run_time_configurable_transform_length=off  phase_factor_width=17  scaling_options=unscaled  rounding_modes=convergent_rounding  aclken=off  aresetn=off  output_ordering=natural_order  cyclic_prefix_insertion=off  throttle_scheme=nonrealtime  xk_index=on  ovflo=off  trim_axipin_name=on  memory_options_data=block_ram  memory_options_phase_factors=block_ram  number_of_stages_using_block_ram_for_data_and_phase_factors=0  memory_options_reorder=block_ram  memory_options_hybrid=off  complex_mult_type=use_mults_resources  butterfly_type=use_xtremedsp_slices  simulation_type=hybrid_sim  simulation_model=sysgen:xfftv9_cmodel  data_path_portlist={ 's_axis_data_tdata', 'm_axis_data_tdata', 'm_axis_status_tdata', 'event_fft_overflow' }  channels=1  input_ordering=natural_order  input_width=16  ip_name=Fast Fourier Transform  ip_version=9.0  dsptool_ready=true  ipcore_usecache=true  ipcore_useipmodelcache=true  wrapper_available=true  port_translation_map={ 'aclken' => 'en', 'aresetn' => 'rst'}  data_format=fixed_point  block_type=xfft_v9_0
  IFFT : xbsIndex_r4/Constant  const=0  gui_display_data_type=Fixed-point  arith_type=Unsigned  n_bits=1  bin_pt=0  preci_type=Single  exp_width=8  frac_width=24  explicit_period=off  period=1  equ=P=C  opselect=C  inp2=PCIN>>17  opr=+  inp1=P  carry=CIN  dbl_ovrd=off  block_type=constant
  IFFT1 : xbsIndex_r4/Constant  const=0  gui_display_data_type=Fixed-point  arith_type=Unsigned  n_bits=1  bin_pt=0  preci_type=Single  exp_width=8  frac_width=24  explicit_period=off  period=1  equ=P=C  opselect=C  inp2=PCIN>>17  opr=+  inp1=P  carry=CIN  dbl_ovrd=off  block_type=constant
  Logical : xbsIndex_r4/Logical  logical_function=AND  inputs=2  en=off  latency=1  precision=Full  arith_type=Unsigned  n_bits=16  bin_pt=0  align_bp=on  dbl_ovrd=off  block_type=logical
  Logical1 : xbsIndex_r4/Logical  logical_function=AND  inputs=2  en=off  latency=1  precision=Full  arith_type=Unsigned  n_bits=16  bin_pt=0  align_bp=on  dbl_ovrd=off  block_type=logical
  Logical2 : xbsIndex_r4/Logical  logical_function=AND  inputs=2  en=off  latency=0  precision=Full  arith_type=Unsigned  n_bits=16  bin_pt=0  align_bp=on  dbl_ovrd=off  block_type=logical
  Logical3 : xbsIndex_r4/Logical  logical_function=AND  inputs=2  en=off  latency=0  precision=Full  arith_type=Unsigned  n_bits=16  bin_pt=0  align_bp=on  dbl_ovrd=off  block_type=logical
  Logical4 : xbsIndex_r4/Logical  logical_function=AND  inputs=2  en=off  latency=1  precision=Full  arith_type=Unsigned  n_bits=16  bin_pt=0  align_bp=on  dbl_ovrd=off  block_type=logical
  ROM1 : xbsIndex_r4/ROM  depth=8  initVector=imag(exp(j*2*pi*(0:7)/16))  distributed_mem=Block RAM  rst=off  init_reg=0  en=off  latency=1  gui_display_data_type=Fixed-point  arith_type="Signed  (2's comp)"  n_bits=18  bin_pt=17  preci_type=Single  exp_width=8  frac_width=24  optimize=Area  use_rpm=on  dbl_ovrd=off  block_type=sprom
  ROM2 : xbsIndex_r4/ROM  depth=8  initVector=real(exp(j*2*pi*(0:7)/16))  distributed_mem=Block RAM  rst=off  init_reg=0  en=off  latency=1  gui_display_data_type=Fixed-point  arith_type="Signed  (2's comp)"  n_bits=18  bin_pt=17  preci_type=Single  exp_width=8  frac_width=24  optimize=Area  use_rpm=on  dbl_ovrd=off  block_type=sprom
  Register{,1..7} (8 alike) : xbsIndex_r4/Register  init=0  rst=off  en=off  dbl_ovrd=off  block_type=register
  Relational : xbsIndex_r4/Relational  mode=a=b  op_type=Bool  en=off  latency=1  dbl_ovrd=off  block_type=relational
  Scale{,1..3} (4 alike) : xbsIndex_r4/Scale  scale_factor=-1  dbl_ovrd=off  block_type=scale
  concat1 : xbsIndex_r4/BitBasher  bitexpr=o={21'b0,index, im[19:0], re[19:0] }  display_expr=off  sr_1=o  arith_type1=Unsigned  bin_pt1=0  sr_2=2  arith_type2=Unsigned  bin_pt2=0  sr_3=3  arith_type3=Unsigned  bin_pt3=0  sr_4=4  arith_type4=Unsigned  bin_pt4=0  dbl_ovrd=off  block_type=bitbasher
  concat2 : xbsIndex_r4/BitBasher  bitexpr=o={21'b0,index, im[19:0], re[19:0] }  display_expr=off  sr_1=o  arith_type1=Unsigned  bin_pt1=0  sr_2=2  arith_type2=Unsigned  bin_pt2=0  sr_3=3  arith_type3=Unsigned  bin_pt3=0  sr_4=4  arith_type4=Unsigned  bin_pt4=0  dbl_ovrd=off  block_type=bitbasher
  concat3 : xbsIndex_r4/BitBasher  bitexpr=o={hi,low }  display_expr=off  sr_1=o  arith_type1=Unsigned  bin_pt1=0  sr_2=2  arith_type2=Unsigned  bin_pt2=0  sr_3=3  arith_type3=Unsigned  bin_pt3=0  sr_4=4  arith_type4=Unsigned  bin_pt4=0  dbl_ovrd=off  block_type=bitbasher
  concat4 : xbsIndex_r4/BitBasher  bitexpr=o={hi,low }  display_expr=off  sr_1=o  arith_type1=Unsigned  bin_pt1=0  sr_2=2  arith_type2=Unsigned  bin_pt2=0  sr_3=3  arith_type3=Unsigned  bin_pt3=0  sr_4=4  arith_type4=Unsigned  bin_pt4=0  dbl_ovrd=off  block_type=bitbasher
  imag0 : xbsIndex_r4/Register  init=0  rst=off  en=off  dbl_ovrd=off  block_type=register
  imag1 : xbsIndex_r4/Register  init=0  rst=off  en=off  dbl_ovrd=off  block_type=register
  real0 : xbsIndex_r4/Register  init=0  rst=off  en=off  dbl_ovrd=off  block_type=register
  real1 : xbsIndex_r4/Register  init=0  rst=off  en=off  dbl_ovrd=off  block_type=register
  split1 : xbsIndex_r4/BitBasher  bitexpr=|  display_expr=off  sr_1=re  arith_type1="Signed  (2's comp)"  bin_pt1=13  sr_2=im  arith_type2="Signed  (2's comp)"  bin_pt2=13  sr_3=index  arith_type3=Unsigned  bin_pt3=0  sr_4=4  arith_type4=Unsigned  bin_pt4=0  dbl_ovrd=off  block_type=bitbasher
      | re={in[19:2]}
      | im={in[39:22]}
      | index = {in[42:40]}
  split2 : xbsIndex_r4/BitBasher  bitexpr=|  display_expr=off  sr_1=re  arith_type1="Signed  (2's comp)"  bin_pt1=13  sr_2=im  arith_type2="Signed  (2's comp)"  bin_pt2=13  sr_3=index  arith_type3=Unsigned  bin_pt3=0  sr_4=4  arith_type4=Unsigned  bin_pt4=0  dbl_ovrd=off  block_type=bitbasher
      | re={in[19:2]}
      | im={in[39:22]}
      | index = {in[42:40]}
  tlast2 : xbsIndex_r4/Constant  const=0  gui_display_data_type=Boolean  arith_type=Boolean  n_bits=8  bin_pt=0  preci_type=Single  exp_width=8  frac_width=24  explicit_period=off  period=1  equ=P=C  opselect=C  inp2=PCIN>>17  opr=+  inp1=P  carry=CIN  dbl_ovrd=off  block_type=constant
  tlast3 : xbsIndex_r4/Constant  const=0  gui_display_data_type=Boolean  arith_type=Boolean  n_bits=8  bin_pt=0  preci_type=Single  exp_width=8  frac_width=24  explicit_period=off  period=1  equ=P=C  opselect=C  inp2=PCIN>>17  opr=+  inp1=P  carry=CIN  dbl_ovrd=off  block_type=constant
  valid : xbsIndex_r4/Register  init=0  rst=off  en=off  dbl_ovrd=off  block_type=register
  valid_o : Outport
  im0 : Outport  Port=2
  re0 : Outport  Port=3
  ready_i : Outport  Port=4
  wires:
  Convert5/1 -> concat4/2
  Convert1/1 -> concat4/1
  Register7/1 -> Convert2/1
  Register6/1 -> Convert3/1
  Register5/1 -> Fast Fourier Transform 9.0 2/6, Fast Fourier Transform 9.0 1/6
  Register4/1 -> Fast Fourier Transform 9.0 2/5
  Logical4/1 -> Fast Fourier Transform 9.0 1/5
  Register3/1 -> BitBasher1/1
  AXI FIFO2/2 -> Register3/1
  BitBasher1/2 -> Fast Fourier Transform 9.0 1/4
  BitBasher1/1 -> Fast Fourier Transform 9.0 1/3
  AXI FIFO2/1 -> Logical4/2
  BitBasher/1 -> AXI FIFO2/3
  Scale1/1 -> BitBasher/2
  Scale/1 -> BitBasher/1
  Delay11/1 -> imag0/1
  Delay10/1 -> imag1/1
  Delay9/1 -> real0/1
  Delay7/1 -> real1/1
  AXI FIFO1/3 -> Fast Fourier Transform 9.0 2/7
  Fast Fourier Transform 9.0 1/1 -> Fast Fourier Transform 9.0 1/2
  Fast Fourier Transform 9.0 2/1 -> Fast Fourier Transform 9.0 2/2
  "Complex Multiplier 6.0 "/2 -> Register5/1
  Constant/1 -> Relational/2
  Relational/1 -> "Complex Multiplier 6.0 "/2
  ROM1/1 -> "Complex Multiplier 6.0 "/6
  ROM2/1 -> "Complex Multiplier 6.0 "/7
  Register1/1 -> "Complex Multiplier 6.0 "/3
  Register/1 -> "Complex Multiplier 6.0 "/4
  "Complex Multiplier 6.0 "/4 -> Register7/1
  "Complex Multiplier 6.0 "/3 -> Register6/1
  Scale3/1 -> Register/1
  Scale2/1 -> Register1/1
  valid_i/1 -> valid/1
  real_i1/1 -> Delay7/1
  real_i0/1 -> Delay9/1
  imag_i1/1 -> Delay10/1
  imag_i0/1 -> Delay11/1
  split1/3 -> FIR Compiler 7.2 1/6
  split2/3 -> FIR Compiler 7.2 2/6
  tlast3/1 -> FIR Compiler 7.2 1/5
  tlast2/1 -> FIR Compiler 7.2 2/5
  Logical2/1 -> FIR Compiler 7.2 1/1, FIR Compiler 7.2 1/4
  split1/2 -> FIR Compiler 7.2 1/3
  Logical3/1 -> FIR Compiler 7.2 2/1, FIR Compiler 7.2 2/4
  split2/2 -> FIR Compiler 7.2 2/3
  Fast Fourier Transform 9.0 2/4 -> concat2/3
  split1/1 -> FIR Compiler 7.2 1/2
  FIR Compiler 7.2 2/5 -> Convert6/1
  FIR Compiler 7.2 2/4 -> Convert5/1
  FIR Compiler 7.2 1/5 -> Convert4/1
  FIR Compiler 7.2 1/4 -> Convert1/1
  AXI FIFO1/1 -> Logical3/2
  AXI FIFO/1 -> Logical2/2
  AddSub/1 -> Scale/1
  Fast Fourier Transform 9.0 1/5 -> concat1/2
  AXI FIFO/2 -> split1/1
  concat2/1 -> AXI FIFO1/3
  Fast Fourier Transform 9.0 2/6 -> AXI FIFO1/2
  Fast Fourier Transform 9.0 2/5 -> concat2/2
  Fast Fourier Transform 9.0 2/3 -> concat2/1
  Fast Fourier Transform 9.0 1/4 -> concat1/3
  Fast Fourier Transform 9.0 1/6 -> AXI FIFO/2
  Delay4/1 -> Register2/1, Counter/1, AXI FIFO2/2
  "Complex Multiplier 6.0 "/1 -> Logical4/1, AXI FIFO2/1, Register4/1
  Convert2/1 -> Fast Fourier Transform 9.0 2/4
  Counter/1 -> ROM1/1, Relational/1, ROM2/1
  Logical1/1 -> valid_o/1
  FIR Compiler 7.2 2/3 -> Logical1/2
  FIR Compiler 7.2 1/3 -> Logical1/1
  AddSub2/1 -> Scale2/1
  AddSub4/1 -> Scale3/1
  imag0/1 -> AddSub/1, AddSub2/1
  valid/1 -> Delay4/1
  real1/1 -> AddSub1/2, AddSub4/2
  imag1/1 -> AddSub/2, AddSub2/2
  real0/1 -> AddSub1/1, AddSub4/1
  Logical/1 -> ready_i/1
  Fast Fourier Transform 9.0 2/2 -> Logical/1
  Fast Fourier Transform 9.0 1/2 -> Logical/2
  AddSub1/1 -> Scale1/1
  FIR Compiler 7.2 2/1 -> AXI FIFO1/1, Logical3/1
  split2/1 -> FIR Compiler 7.2 2/2
  FIR Compiler 7.2 1/1 -> AXI FIFO/1, Logical2/1
  AXI FIFO1/2 -> split2/1
  Register2/1 -> "Complex Multiplier 6.0 "/5, "Complex Multiplier 6.0 "/1
  Convert3/1 -> Fast Fourier Transform 9.0 2/3
  IFFT1/1 -> Fast Fourier Transform 9.0 2/1
  AXI FIFO/3 -> Fast Fourier Transform 9.0 1/7
  concat1/1 -> AXI FIFO/3
  Fast Fourier Transform 9.0 1/3 -> concat1/1
  IFFT/1 -> Fast Fourier Transform 9.0 1/1
  concat4/1 -> re0/1
  Convert4/1 -> concat3/1
  Convert6/1 -> concat3/2
  concat3/1 -> im0/1

== system sysgen_oversample2x_2samples_per_clock/analysis_sysgen/Analysis0/channel_select1 ==
  tready : Inport
  data_valid : Inport  Port=2
  Constant : xbsIndex_r4/Constant  const=6  gui_display_data_type=Fixed-point  arith_type=Unsigned  n_bits=3  bin_pt=0  preci_type=Single  exp_width=8  frac_width=24  explicit_period=off  period=1  equ=P=C  opselect=C  inp2=PCIN>>17  opr=+  inp1=P  carry=CIN  dbl_ovrd=off  block_type=constant
  Counter : xbsIndex_r4/Counter  cnt_type=Free Running  cnt_to=Inf  operation=Up  start_count=0  cnt_by_val=1  arith_type=Unsigned  n_bits=3  bin_pt=0  load_pin=off  rst=off  en=on  explicit_period=on  period=2  use_behavioral_HDL=off  implementation=Fabric  dbl_ovrd=off  block_type=counter
  Logical6 : xbsIndex_r4/Logical  logical_function=AND  inputs=2  en=off  latency=1  precision=Full  arith_type=Unsigned  n_bits=16  bin_pt=0  align_bp=on  dbl_ovrd=off  block_type=logical
  Relational : xbsIndex_r4/Relational  mode=a=b  op_type=Bool  en=off  latency=1  dbl_ovrd=off  block_type=relational
  tvalid : Outport
  tdata_fsel : Outport  Port=2
  t_last : Outport  Port=3
  wires:
  Logical6/1 -> tvalid/1, Counter/1
  data_valid/1 -> Logical6/2
  Counter/1 -> Relational/2, tdata_fsel/1
  tready/1 -> Logical6/1
  Relational/1 -> t_last/1
  Constant/1 -> Relational/1

== system sysgen_oversample2x_2samples_per_clock/analysis_sysgen/Analysis2/channel_select1 ==
  tready : Inport
  data_valid : Inport  Port=2
  Constant : xbsIndex_r4/Constant  const=6  gui_display_data_type=Fixed-point  arith_type=Unsigned  n_bits=3  bin_pt=0  preci_type=Single  exp_width=8  frac_width=24  explicit_period=off  period=1  equ=P=C  opselect=C  inp2=PCIN>>17  opr=+  inp1=P  carry=CIN  dbl_ovrd=off  block_type=constant
  Counter : xbsIndex_r4/Counter  cnt_type=Free Running  cnt_to=Inf  operation=Up  start_count=0  cnt_by_val=1  arith_type=Unsigned  n_bits=3  bin_pt=0  load_pin=off  rst=off  en=on  explicit_period=on  period=2  use_behavioral_HDL=off  implementation=Fabric  dbl_ovrd=off  block_type=counter
  Logical6 : xbsIndex_r4/Logical  logical_function=AND  inputs=2  en=off  latency=1  precision=Full  arith_type=Unsigned  n_bits=16  bin_pt=0  align_bp=on  dbl_ovrd=off  block_type=logical
  Relational : xbsIndex_r4/Relational  mode=a=b  op_type=Bool  en=off  latency=1  dbl_ovrd=off  block_type=relational
  tvalid : Outport
  tdata_fsel : Outport  Port=2
  t_last : Outport  Port=3
  wires:
  Constant/1 -> Relational/1
  Relational/1 -> t_last/1
  tready/1 -> Logical6/1
  Counter/1 -> tdata_fsel/1, Relational/2
  data_valid/1 -> Logical6/2
  Logical6/1 -> Counter/1, tvalid/1
